simulink model "Masseschwinger_Variabel"  (R2026a)
settings: Solver=ode3  StopTime=30  FixedStep=0.0001
settings Model: Creator=alfa  LastModifiedBy=alfa

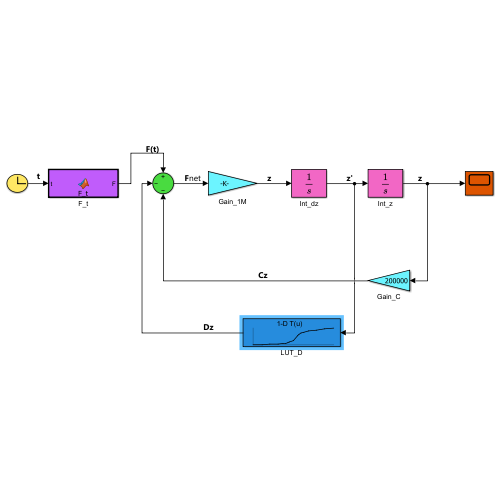
[thumbnail: Simulink's stored preview of the top-level diagram]
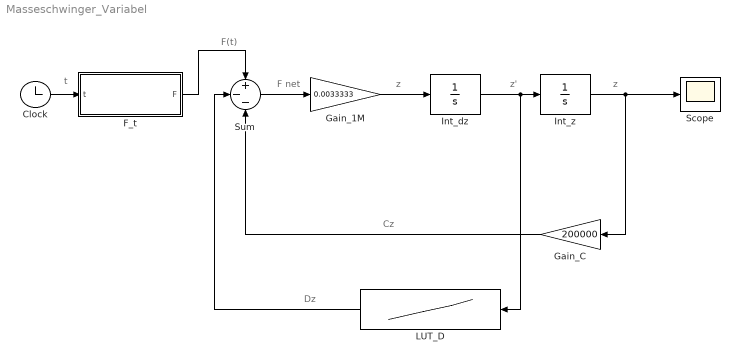
== system Masseschwinger_Variabel ==
  note: t
  note: F net
  note: F(t)
  note: z
  note: Dz
  note: Cz
  note: z'
  note: z
  Clock : Clock
  F_t : MATLAB Function  TreatAsAtomicUnit=on
  Gain_1M : Gain  Gain=0.0033333
  Gain_C : Gain  Gain=200000
  Int_dz : Integrator
  Int_z : Integrator
  LUT_D : Lookup_n-D  NumberOfTableDimensions=1  BreakpointsForDimension1=[-0.52 -0.4 -0.3 -0.2 -0.13 -0.1 -0.075 -0.05 0 0.05 0.075 0.1 0.13 0.2 0.3 0.4 0.52]  Table=[-433 -400 -367 -325 -285 -257 -220 -133 0 500 660 770 855 975 1100 1200 1300]  InternalRulePriority=Speed  RndMeth=Simplest
  Scope : Scope
      settings: ActiveDisplayYMinimum=-0.0013387619530462109  ActiveDisplayYMaximum=0.0067011390694647933
  Sum : Sum  Inputs=+--
  wires:
  F_t/1(F) -> Sum/1
  Sum/1 -> Gain_1M/1
  Gain_1M/1 -> Int_dz/1
  Int_dz/1 -> Int_z/1, LUT_D/1
  Int_z/1 -> Scope/1, Gain_C/1
  Clock/1 -> F_t/1(t)
  Gain_C/1 -> Sum/3
  LUT_D/1 -> Sum/2

== matlab function Masseschwinger_Variabel/F_t ==
  data: t input; F output
function F = F_t(t)
  H = 1111.0;
  omega = 0.90;
  F = 0.5*H*(t>=3) + H*((t>=1)-(t>=3))*sin(omega*t);
end
